simulink library "rocket_data_library"  (R2014a)
settings: Solver=ode45  StartTime=0.0  StopTime=10.0  RelTol=1e-3
settings Model: Creator=scorpii  LastModifiedBy=scorpii

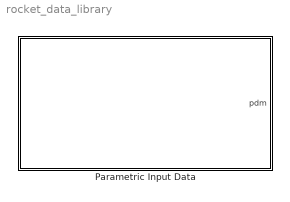
== system rocket_data_library ==
  Parametric Input Data : Subsystem

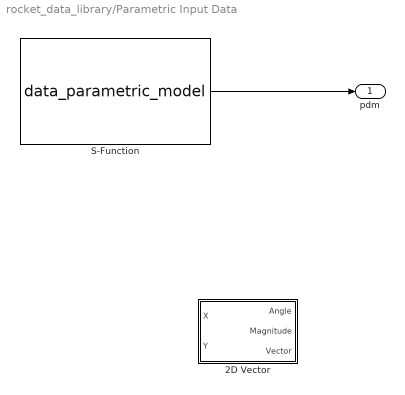
== system rocket_data_library/Parametric Input Data ==
  2D Vector : Subsystem
  S-Function : S-Function  FunctionName=data_parametric_model  Parameters=pdm  EnableBusSupport=off
  pdm : Outport
  wires:
  S-Function/1 -> pdm/1

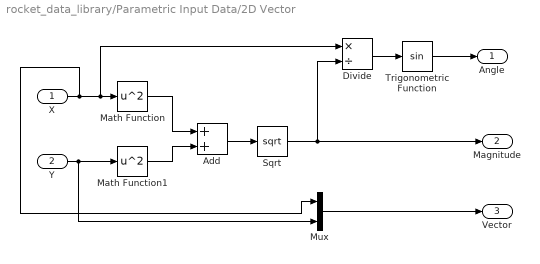
== system rocket_data_library/Parametric Input Data/2D Vector ==
  X : Inport
  Y : Inport  Port=2
  Add : Sum
  Divide : Product  Inputs=*/
  Math Function : Math  Operator=square  SaturateOnIntegerOverflow=on
  Math Function1 : Math  Operator=square  SaturateOnIntegerOverflow=on
  Mux : Mux  Inputs=2
  Sqrt : Sqrt  SaturateOnIntegerOverflow=on
  Trigonometric Function : Trigonometry
  Angle : Outport
  Magnitude : Outport  Port=2
  Vector : Outport  Port=3
  wires:
  Trigonometric Function/1 -> Angle/1
  Add/1 -> Sqrt/1
  Sqrt/1 -> Magnitude/1, Divide/2
  Math Function1/1 -> Add/2
  Y/1 -> Mux/2, Math Function1/1
  Math Function/1 -> Add/1
  Divide/1 -> Trigonometric Function/1
  X/1 -> Mux/1, Divide/1, Math Function/1
  Mux/1 -> Vector/1
